simulink model "GEARBOX_OTLADKA"  (R2023a)
settings: Solver=VariableStepAuto  StartTime=0.0  StopTime=1  RelTol=1e-3
settings Model: Creator=ycheb  LastModifiedBy=ycheb

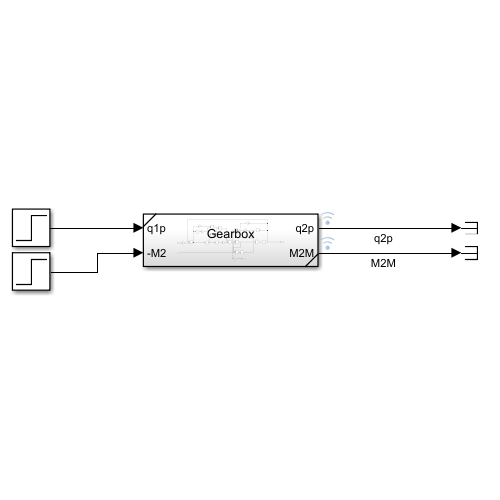
[thumbnail: Simulink's stored preview of the top-level diagram]
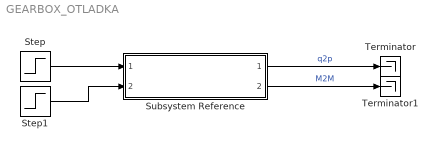
== system GEARBOX_OTLADKA ==
  Step : Step  Time=0  SampleTime=0
  Step1 : Step  Time=0  SampleTime=0
  Subsystem Reference : Subsystem  ReferencedSubsystem=Gearbox
  Terminator : Terminator
  Terminator1 : Terminator
  wires:
  Step1/1 -> Subsystem Reference/2
  Step/1 -> Subsystem Reference/1
  Subsystem Reference/2 -> Terminator1/1  "M2M"
  Subsystem Reference/1 -> Terminator/1  "q2p"
